simulink model "sample1_cw_acw1_signal"  (R2021b)
settings: Solver=FixedStepDiscrete  StartTime=0.0  StopTime=255*2  FixedStep=1  RelTol=1e-3
libraries: simulink x1
settings Model: Creator=kawata  LastModifiedBy=kawata
settings DataIOCC: ReturnWorkspaceOutputs=off

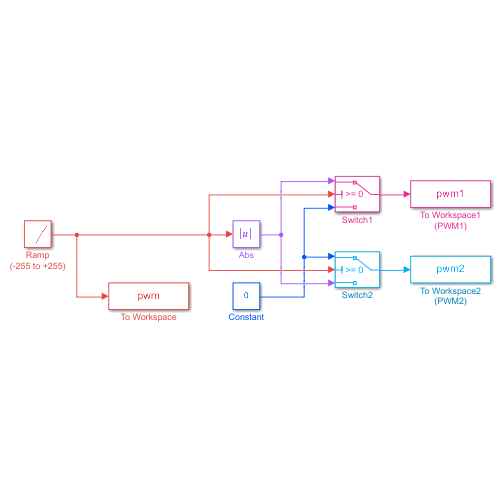
[thumbnail: Simulink's stored preview of the top-level diagram]
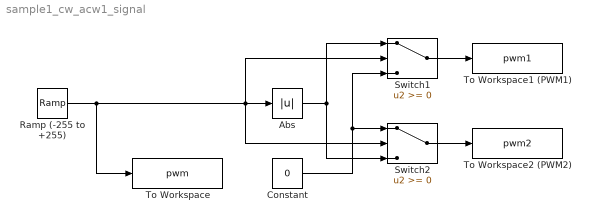
== system sample1_cw_acw1_signal ==
  Abs : Abs
  Constant : Constant  Value=0
  Ramp (-255 to +255) : simulink/Sources/Ramp  slope=1  start=0  InitialOutput=-255
  Switch1 : Switch
  Switch2 : Switch
  To Workspace : ToWorkspace  VariableName=pwm  SampleTime=-1
  To Workspace1 (PWM1) : ToWorkspace  VariableName=pwm1  SampleTime=-1
  To Workspace2 (PWM2) : ToWorkspace  VariableName=pwm2  SampleTime=-1
  wires:
  Abs/1 -> Switch2/3, Switch1/1
  Ramp (-255 to +255)/1 -> Abs/1, Switch1/2, Switch2/2, To Workspace/1
  Constant/1 -> Switch1/3, Switch2/1
  Switch1/1 -> To Workspace1 (PWM1)/1
  Switch2/1 -> To Workspace2 (PWM2)/1
